simulink model "BLAC0_v1_simulink"  (R2018b)
settings: Solver=VariableStepAuto  StartTime=0.0  StopTime=10.0  RelTol=1e-3
values from neighbouring files (symbols this model uses):
  B = 3.8e-005    (= 3.8e-05)    [BLAC0_v1.m]    (also in BLAC1_v1.m = 0; BLAC1_v2.m = 0; CAE_11_v_1.m = 0; CAE_14_v1.M = 0)
  Crn = 0.6    [BLAC0_v1.m]    (also in BLAC1_v1.m; BLAC1_v2.m; CAE_11_v_1.m; CAE_14_v1.M)
  J = 0.0000251    (= 2.51e-05)    [BLAC0_v1.m]    (also in BLAC1_v1.m = 0.001; BLAC1_v2.m = 0.001; CAE_11_v_1.m = 0.001; CAE_14_v1.M = 0.001)
  Kc = ms*np*lambdaf/2    (= 0.27)    [BLAC0_v1.m]    (also in BLAC1_v1.m = 0.6; BLAC1_v2.m = 0.6; CAE_11_v_1.m = 0.6; CAE_14_v1.M = 0.6)
  Lsd = 0.005/2    (= 0.0025)    [BLAC0_v1.m]    (also in BLAC1_v1.m = 0.005; BLAC1_v2.m = 0.005; CAE_11_v_1.m = 0.005; CAE_14_v1.M = 0.005)
  Lsq = Lsd    (= 0.0025)    [BLAC0_v1.m]    (also in BLAC1_v1.m = 0.005; BLAC1_v2.m = 0.005; CAE_11_v_1.m = 0.005; CAE_14_v1.M = 0.005)
  np = 2    [BLAC0_v1.m]    (also in BLAC1_v1.m = 4; BLAC1_v2.m = 4; CAE_11_v_1.m = 4; CAE_14_v1.M = 4)
  PSIPM = lambdaf    (= 0.09)    [BLAC0_v1.m]
  Rs = 3.1/2    (= 1.55)    [BLAC0_v1.m]    (also in BLAC1_v1.m = 1; BLAC1_v2.m = 1; CAE_11_v_1.m = 1; CAE_14_v1.M = 1)
  wrr = 1256.6    [BLAC0_v1.m]    (also in BLAC1_v1.m = 300; BLAC1_v2.m = 300)
settings Model: Creator=anton  LastModifiedBy=anton

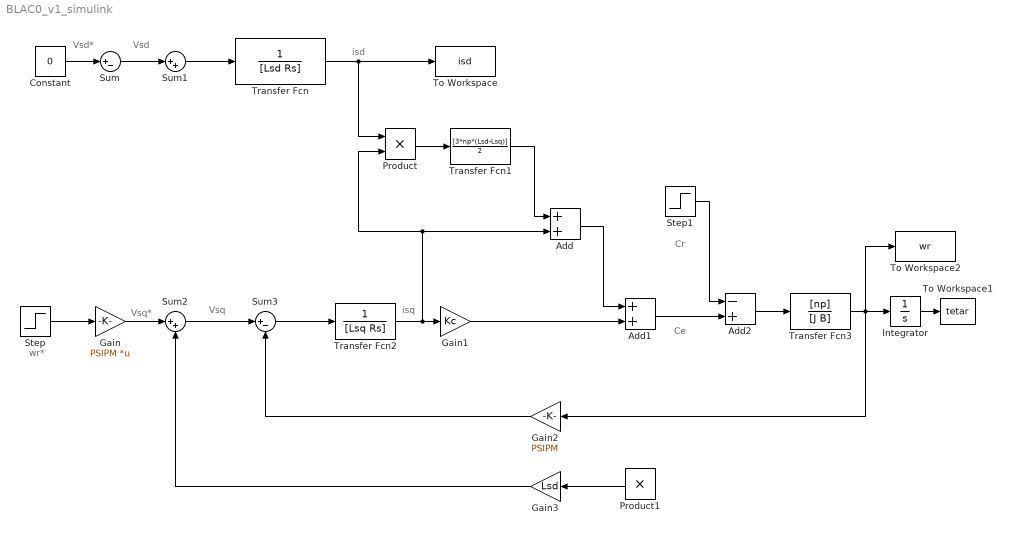
== system BLAC0_v1_simulink ==
  note: Ce
  note: Cr
  note: isq
  note: Vsq
  note: Vsq*
  note: wr*
  note: isd
  note: Vsd
  note: Vsd*
  Add : Sum
  Add1 : Sum
  Add2 : Sum  Inputs=-+
  Constant : Constant  Value=0
  Gain : Gain  Gain=PSIPM  Multiplication=Matrix(K*u)
  Gain1 : Gain  Gain=Kc
  Gain2 : Gain  Gain=PSIPM
  Gain3 : Gain  Gain=Lsd
  Integrator : Integrator
  Product : Product
  Product1 : Product
  Step : Step  After=wrr  SampleTime=0
  Step1 : Step  After=Crn  SampleTime=0
  Sum : Sum  Inputs=|+-
  Sum1 : Sum  Inputs=|++
  Sum2 : Sum  Inputs=|++
  Sum3 : Sum  Inputs=|+-
  To Workspace : ToWorkspace  VariableName=isd  SaveFormat=Timeseries  SampleTime=-1
  To Workspace1 : ToWorkspace  VariableName=tetar  SaveFormat=Timeseries  SampleTime=-1
  To Workspace2 : ToWorkspace  VariableName=wr  SaveFormat=Timeseries  SampleTime=-1
  Transfer Fcn : TransferFcn  Denominator=[Lsd Rs]
  Transfer Fcn1 : TransferFcn  Numerator=[3*np*(Lsd-Lsq)]  Denominator=[2]
  Transfer Fcn2 : TransferFcn  Denominator=[Lsq Rs]
  Transfer Fcn3 : TransferFcn  Numerator=[np]  Denominator=[J B]
  wires:
  Constant/1 -> Sum/1
  Sum/1 -> Sum1/1
  Sum1/1 -> Transfer Fcn/1
  Transfer Fcn/1 -> Product/1, To Workspace/1
  Product/1 -> Transfer Fcn1/1
  Transfer Fcn1/1 -> Add/1
  Step/1 -> Gain/1
  Gain/1 -> Sum2/1
  Sum2/1 -> Sum3/1
  Sum3/1 -> Transfer Fcn2/1
  Transfer Fcn2/1 -> Add/2, Product/2, Gain1/1
  Add/1 -> Add1/1
  Gain1/1 -> Add1/2
  Add1/1 -> Add2/2
  Step1/1 -> Add2/1
  Add2/1 -> Transfer Fcn3/1
  Transfer Fcn3/1 -> Gain2/1, To Workspace2/1, Integrator/1
  Integrator/1 -> To Workspace1/1
  Gain2/1 -> Sum3/2
  Gain3/1 -> Sum2/2
  Product1/1 -> Gain3/1
